simulink subsystem "Mechanical_part"  (R2023a)
settings: Solver=VariableStepAuto  StartTime=0.0  StopTime=10.0  RelTol=1e-3
model mask{C_M=C_M, J_m=J_m}
  mask prompts: C_M "Mechanical coef"; J_m "Motor inertion"
settings Model: Creator=ПК  LastModifiedBy=ПК

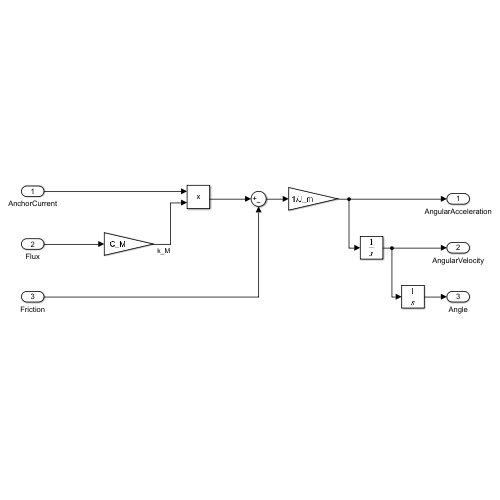
[thumbnail: Simulink's stored preview of the top-level diagram]
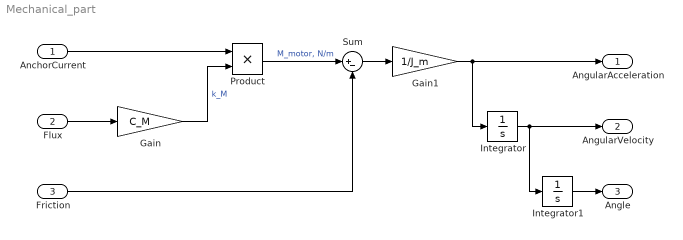
== system Mechanical_part ==
  AnchorCurrent : Inport
  Flux : Inport  Port=2
  Friction : Inport  Port=3
  Gain : Gain  Gain=C_M
  Gain1 : Gain  Gain=1/J_m
  Integrator : Integrator
  Integrator1 : Integrator
  Product : Product
  Sum : Sum  Inputs=|+-
  AngularAcceleration : Outport
  AngularVelocity : Outport  Port=2
  Angle : Outport  Port=3
  wires:
  AnchorCurrent/1 -> Product/1
  Gain/1 -> Product/2  "k_M"
  Flux/1 -> Gain/1
  Friction/1 -> Sum/2
  Product/1 -> Sum/1  "M_motor, N/m"
  Sum/1 -> Gain1/1
  Gain1/1 -> Integrator/1, AngularAcceleration/1
  Integrator/1 -> Integrator1/1, AngularVelocity/1
  Integrator1/1 -> Angle/1
